simulink model "management_2_sources_21_03_2023_flc_9aa"  (R2016b)
settings: Solver=FixedStepAuto  StartTime=0.0  StopTime=25  RelTol=1e-3
undefined symbols (not defined in the file): DiscIntNeverNeededParam, sigbuilder_block
libraries: powerlib x31, simulink x8, powerlib_meascontrol x7, fuzblock x1, powerlib_extras x1
(part 2 of 2)

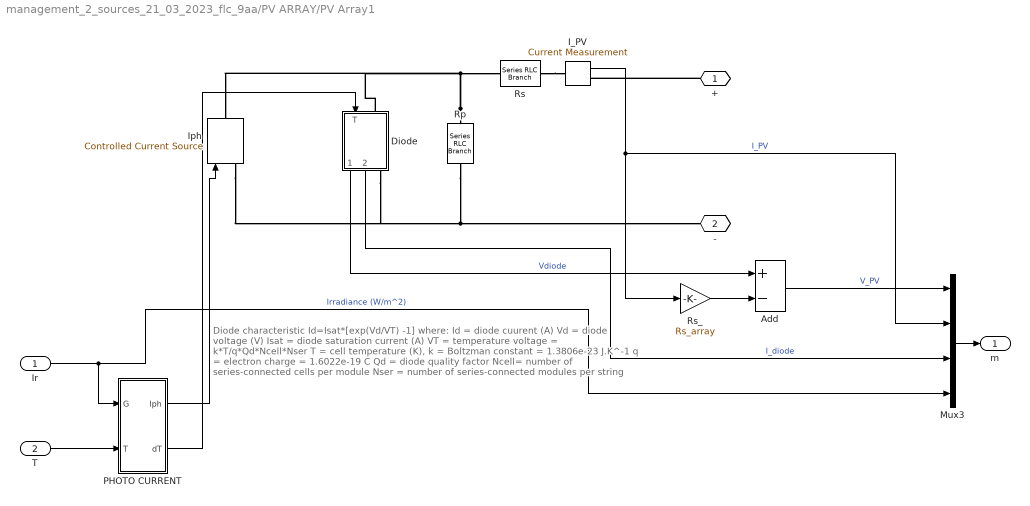
== system management_2_sources_21_03_2023_flc_9aa/PV ARRAY/PV Array1 ==
  note: Diode characteristic
      |    Id=Isat*[exp(Vd/VT) -1]
      |
      | where:
      |    Id = diode cuurent (A)
      |    Vd = diode voltage (V)
      |  Isat = diode saturation current (A)
      |    VT = temperature voltage = k*T/q*Qd*Ncell*Nser
      |
      |     T = cell temperature (K),
      |     k = Boltzman constant = 1.3806e-23 J.K^-1
      |     q = electron charge = 1.6022e-19 C
      |    Qd = diode quality factor
      |  Ncell= number of series-connected cells per module
      |  Nser = number of series-connected modules per string
  Ir : Inport
  T : Inport  Port=2
  Add : Sum  Inputs=+-
  Diode : Subsystem
      mask Display:
      | plot(-75,-50,100,150, [-15 -15 43 -15 -15 -75],[50 8 50 92 50 50], ...
      |     [43 43],[8 94],[100 43], [50 50])
  I_PV : powerlib/Measurements/Current Measurement  PhasorSimulation=off  OutputType=Complex  PSBequivalent=0
  Iph : powerlib/Electrical Sources/Controlled Current Source  Initialize=on  Source_Type=AC  Amplitude=0  Phase=0  Frequency=0  Measurements=None
  Mux3 : Mux
  PHOTO CURRENT : Subsystem
  Rp : powerlib/Elements/Series RLC Branch  LConnTagsString=__new0  RConnTagsString=__new0  BranchType=R  Resistance=Rp_array  Inductance=1e-3  SetiL0=off  InitialCurrent=0  Capacitance=1e-6  Setx0=off  InitialVoltage=0  Measurements=Branch current
  Rs : powerlib/Elements/Series RLC Branch  LConnTagsString=__new0  RConnTagsString=__new0  BranchType=R  Resistance=Rs_array  Inductance=1e-3  SetiL0=off  InitialCurrent=0  Capacitance=1e-6  Setx0=off  InitialVoltage=0  Measurements=None
  Rs_ : Gain  Gain=Rs_array
  + : PMIOPort  Port=1  Side=Right
  - : PMIOPort  Port=2  Side=Right
  m : Outport
  wires:
  Diode/2(Idiode) -> Mux3/3  "I_diode"
  Add/1 -> Mux3/1  "V_PV"
  I_PV/1 -> Mux3/2, Rs_/1  "I_PV"
  Rs_/1 -> Add/2
  Diode/1(Vdiode) -> Add/1  "Vdiode"
  Ir/1 -> Mux3/4, PHOTO CURRENT/1(G)  "Irradiance (W/m^2)"
  PHOTO CURRENT/1("Iph ") -> Iph/1
  T/1 -> PHOTO CURRENT/2(T)
  PHOTO CURRENT/2(dT) -> Diode/1(T)
  Mux3/1 -> m/1
  connections:
  +/RConn1 -- I_PV/RConn1
  Rs/LConn1 -- I_PV/LConn1
  Rp/LConn1 -- Rs/RConn1 -- Iph/RConn1 -- Diode/LConn1
  Rp/RConn1 -- -/RConn1 -- Diode/RConn1 -- Iph/LConn1

== system management_2_sources_21_03_2023_flc_9aa/PV ARRAY/boost converter ==
  pwm : Inport
  C1 : powerlib/Elements/Series RLC Branch  LConnTagsString=__new0  RConnTagsString=__new0  BranchType=C  Resistance=1.0  Inductance=1.0  SetiL0=off  InitialCurrent=0  Capacitance=100e-6  Setx0=off  InitialVoltage=0  Measurements=None
  Diode1 : powerlib/Power Electronics/Diode  Ron=1e-4  Lon=0  Vf=0  IC=0  UseSnubber=off  Rs=inf  Cs=inf  Measurements=off
  IGBT1 : powerlib/Power Electronics/IGBT  Ron=0.001  Lon=0  Vf=0  Tf=0  Tt=0  IC=0  Rs=1e5  Cs=inf  Measurements=off
  L1 : powerlib/Elements/Series RLC Branch  LConnTagsString=__new0  RConnTagsString=__new0  BranchType=RL  Resistance=0.005  Inductance=5e-3  SetiL0=off  InitialCurrent=0  Capacitance=1e-6  Setx0=off  InitialVoltage=0  Measurements=None
  out + : PMIOPort  Port=1  Side=Right
  in + : PMIOPort  Port=2  Side=Left
  in - : PMIOPort  Port=3  Side=Left
  out - : PMIOPort  Port=4  Side=Right
  wires:
  pwm/1 -> IGBT1/1
  connections:
  C1/LConn1 -- in +/RConn1 -- L1/LConn1
  IGBT1/LConn1 -- L1/RConn1 -- Diode1/LConn1
  out +/RConn1 -- Diode1/RConn1
  C1/RConn1 -- in -/RConn1 -- out -/RConn1 -- IGBT1/RConn1

== system management_2_sources_21_03_2023_flc_9aa/Subsystem2/Dashboard Scope ==

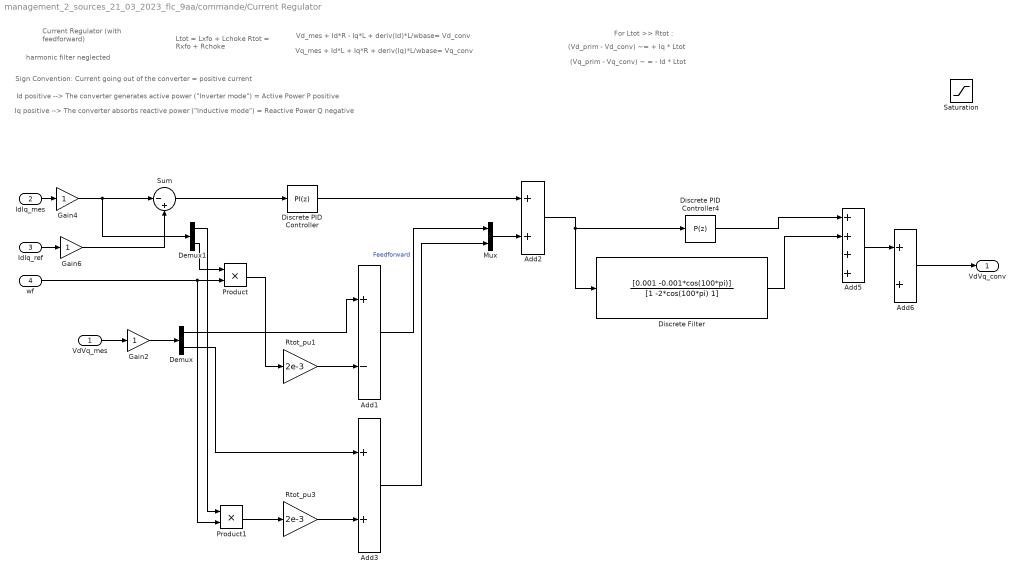
== system management_2_sources_21_03_2023_flc_9aa/commande/Current Regulator ==
  note: harmonic filter neglected
  note: Vd_mes + Id*R - Iq*L + deriv(Id)*L/wbase= Vd_conv
  note: Vq_mes + Id*L + Iq*R + deriv(Iq)*L/wbase= Vq_conv
  note: Current Regulator
      | (with feedforward)
  note: Sign Convention: Current going out of the converter = positive current
  note: Iq positive --> The converter absorbs reactive power ("Inductive mode") = Reactive Power Q negative
  note: Id positive --> The converter generates active power ("Inverter mode") = Active Power P positive
  note: Ltot = Lxfo + Lchoke
      | Rtot = Rxfo + Rchoke
  note: (Vd_prim - Vd_conv) ~= + Iq * Ltot
  note: (Vq_prim - Vq_conv) ~ = - Id * Ltot
  note: For Ltot >> Rtot :
  VdVq_mes : Inport  PortDimensions=2
  IdIq_mes : Inport  Port=2  PortDimensions=2
  IdIq_ref : Inport  Port=3  PortDimensions=2
  wf : Inport  Port=4  PortDimensions=1
  Add1 : Sum  Inputs=+-
  Add2 : Sum
  Add3 : Sum
  Add5 : Sum  Inputs=++++
  Add6 : Sum
  Demux : Demux  Outputs=2
  Demux1 : Demux  Outputs=2
  Discrete Filter : DiscreteFilter  Numerator=[0.001 -0.001*cos(100*pi)]  Denominator=[1 -2*cos(100*pi) 1]  SampleTime=1e-5
  Discrete PID Controller : simulink/Continuous/PID Controller  Controller=PI  TimeDomain=Discrete-time  SampleTime=-1  IntegratorMethod=Trapezoidal  FilterMethod=Forward Euler  Form=Parallel  UseFilter=on  ControllerParametersSource=internal  P=24  I=12  D=0  N=100  InitialConditionSource=internal  InitialConditionForIntegrator=0  InitialConditionForFilter=0  ExternalReset=none  LimitOutput=on  UpperSaturationLimit=1000  LowerSaturationLimit=-1000  LinearizeAsGain=off  AntiWindupMode=none  Kb=1  TrackingMode=off  Kt=1  PParamMin=[]  PParamMax=[]  IParamMin=[]  IParamMax=[]  DParamMin=[]  DParamMax=[]  NParamMin=[]  NParamMax=[]  KbParamMin=[]  KbParamMax=[]  KtParamMin=[]  KtParamMax=[]  POutMin=[]  POutMax=[]  IOutMin=[]  IOutMax=[]  DOutMin=[]  DOutMax=[]  NOutMin=[]  NOutMax=[]  KbOutMin=[]  KbOutMax=[]  KtOutMin=[]  KtOutMax=[]  IntegratorOutMin=[]  IntegratorOutMax=[]  FilterOutMin=[]  FilterOutMax=[]  SumOutMin=[]  SumOutMax=[]  SumI1OutMin=[]  SumI1OutMax=[]  SumI2OutMin=[]  SumI2OutMax=[]  SumI3OutMin=[]  SumI3OutMax=[]  SumDOutMin=[]  SumDOutMax=[]  SaturationOutMin=[]  SaturationOutMax=[]  IntegratorContinuousStateAttributes=''  IntegratorStateMustResolveToSignalObject=off  IntegratorRTWStateStorageClass=Auto  FilterContinuousStateAttributes=''  FilterStateMustResolveToSignalObject=off  FilterRTWStateStorageClass=Auto  DifferentiatorICPrevScaledInput=0  DifferentiatorOutMin=[]  DifferentiatorOutMax=[]
  Discrete PID Controller4 : simulink/Continuous/PID Controller  Controller=P  TimeDomain=Discrete-time  SampleTime=-1  IntegratorMethod=Trapezoidal  FilterMethod=Forward Euler  Form=Parallel  UseFilter=on  ControllerParametersSource=internal  P=60  I=12  D=0  N=100  InitialConditionSource=internal  InitialConditionForIntegrator=0  InitialConditionForFilter=0  ExternalReset=none  LimitOutput=on  UpperSaturationLimit=1000  LowerSaturationLimit=-1000  LinearizeAsGain=off  AntiWindupMode=none  Kb=1  TrackingMode=off  Kt=1  PParamMin=[]  PParamMax=[]  IParamMin=[]  IParamMax=[]  DParamMin=[]  DParamMax=[]  NParamMin=[]  NParamMax=[]  KbParamMin=[]  KbParamMax=[]  KtParamMin=[]  KtParamMax=[]  POutMin=[]  POutMax=[]  IOutMin=[]  IOutMax=[]  DOutMin=[]  DOutMax=[]  NOutMin=[]  NOutMax=[]  KbOutMin=[]  KbOutMax=[]  KtOutMin=[]  KtOutMax=[]  IntegratorOutMin=[]  IntegratorOutMax=[]  FilterOutMin=[]  FilterOutMax=[]  SumOutMin=[]  SumOutMax=[]  SumI1OutMin=[]  SumI1OutMax=[]  SumI2OutMin=[]  SumI2OutMax=[]  SumI3OutMin=[]  SumI3OutMax=[]  SumDOutMin=[]  SumDOutMax=[]  SaturationOutMin=[]  SaturationOutMax=[]  IntegratorContinuousStateAttributes=''  IntegratorStateMustResolveToSignalObject=off  IntegratorRTWStateStorageClass=Auto  FilterContinuousStateAttributes=''  FilterStateMustResolveToSignalObject=off  FilterRTWStateStorageClass=Auto  DifferentiatorICPrevScaledInput=0  DifferentiatorOutMin=[]  DifferentiatorOutMax=[]
  Gain2 : Gain
  Gain4 : Gain
  Gain6 : Gain
  Mux : Mux  Inputs=2
  Product : Product
  Product1 : Product
  Rtot_pu1 : Gain  Gain=2e-3  SaturateOnIntegerOverflow=on  OutDataTypeStr=Inherit: Same as input  ParamDataTypeStr=Inherit: Same as input
  Rtot_pu3 : Gain  Gain=2e-3  SaturateOnIntegerOverflow=on  OutDataTypeStr=Inherit: Same as input  ParamDataTypeStr=Inherit: Same as input
  Saturation : Saturate  UpperLimit=5  LowerLimit=-5
  Sum : Sum  Inputs=|-+
  VdVq_conv : Outport
  wires:
  Mux/1 -> Add2/2
  IdIq_ref/1 -> Gain6/1
  Add1/1 -> Mux/1  "Feedforward"
  Add3/1 -> Mux/2
  IdIq_mes/1 -> Gain4/1
  Demux/1 -> Add1/1
  Rtot_pu1/1 -> Add1/2
  Demux/2 -> Add3/1
  Rtot_pu3/1 -> Add3/2
  VdVq_mes/1 -> Gain2/1
  Discrete PID Controller/1 -> Add2/1
  Product/1 -> Rtot_pu1/1
  Demux1/2 -> Product/1
  Product1/1 -> Rtot_pu3/1
  Demux1/1 -> Product1/1
  wf/1 -> Product1/2, Product/2
  Gain4/1 -> Demux1/1, Sum/1
  Gain2/1 -> Demux/1
  Gain6/1 -> Sum/2
  Sum/1 -> Discrete PID Controller/1
  Discrete PID Controller4/1 -> Add5/1
  Add5/1 -> Add6/1
  Add2/1 -> Discrete Filter/1, Discrete PID Controller4/1
  Add6/1 -> VdVq_conv/1
  Discrete Filter/1 -> Add5/2

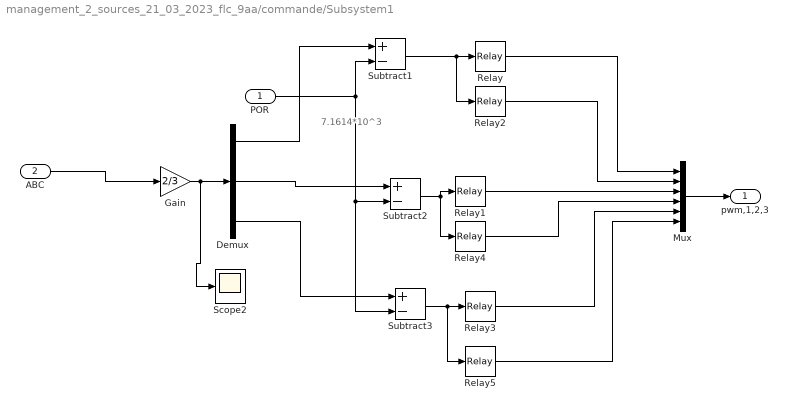
== system management_2_sources_21_03_2023_flc_9aa/commande/Subsystem1 ==
  note: 7.1614*10^3
  POR : Inport
  ABC : Inport  Port=2
  Demux : Demux  Outputs=3
  Gain : Gain  Gain=2/3
  Mux : Mux  Inputs=6
  Relay : Relay
  Relay1 : Relay
  Relay2 : Relay  OnOutputValue=0  OffOutputValue=1
  Relay3 : Relay
  Relay4 : Relay  OnOutputValue=0  OffOutputValue=1
  Relay5 : Relay  OnOutputValue=0  OffOutputValue=1
  Scope2 : Scope
  Subtract1 : Sum  Inputs=+-
  Subtract2 : Sum  Inputs=+-
  Subtract3 : Sum  Inputs=+-
  pwm,1,2,3 : Outport
  wires:
  POR/1 -> Subtract2/2, Subtract3/2, Subtract1/2
  Subtract1/1 -> Relay2/1, Relay/1
  Relay/1 -> Mux/1
  Subtract2/1 -> Relay1/1, Relay4/1
  Mux/1 -> pwm,1,2,3/1
  Gain/1 -> Scope2/1, Demux/1
  Subtract3/1 -> Relay5/1, Relay3/1
  Relay2/1 -> Mux/2
  Relay1/1 -> Mux/3
  Relay4/1 -> Mux/4
  Relay3/1 -> Mux/5
  Relay5/1 -> Mux/6
  Demux/1 -> Subtract1/1
  Demux/2 -> Subtract2/1
  Demux/3 -> Subtract3/1
  ABC/1 -> Gain/1

== system management_2_sources_21_03_2023_flc_9aa/PV ARRAY/Boost Converter Control (MPPT)/Pulse Generator ==
  D : Inport
  Relational Operator : RelationalOperator  Operator=<=  OutDataTypeStr=boolean  RndMeth=Nearest
  Repeating Sequence : simulink/Sources/Repeating Sequence  rep_seq_t="[0  1/Freq]"  rep_seq_y=[0 1]
  Pulses : Outport
  wires:
  D/1 -> Relational Operator/2
  Relational Operator/1 -> Pulses/1
  Repeating Sequence/1 -> Relational Operator/1

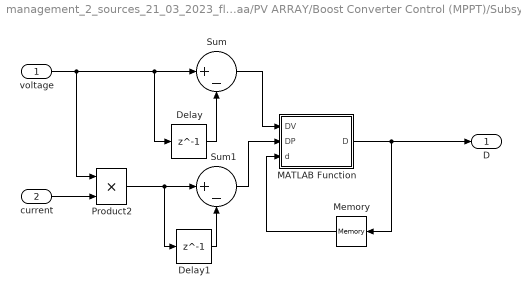
== system management_2_sources_21_03_2023_flc_9aa/PV ARRAY/Boost Converter Control (MPPT)/Subsystem2 ==
  "voltage " : Inport
  "current " : Inport  Port=2
  Delay : Delay  DelayLength=1  InitialCondition=0
  Delay1 : Delay  DelayLength=1  InitialCondition=0
  MATLAB Function : MATLAB Function  TreatAsAtomicUnit=on
  Memory : Memory  X0=0.7
  Product2 : Product
  Sum : Sum  Inputs=|+-
  Sum1 : Sum  Inputs=|+-
  D : Outport
  wires:
  Delay/1 -> Sum/2
  Delay1/1 -> Sum1/2
  "voltage "/1 -> Product2/1, Delay/1, Sum/1
  "current "/1 -> Product2/2
  Sum1/1 -> MATLAB Function/2(DP)
  Sum/1 -> MATLAB Function/1(DV)
  Product2/1 -> Delay1/1, Sum1/1
  MATLAB Function/1(D) -> Memory/1, D/1
  Memory/1 -> MATLAB Function/3(d)

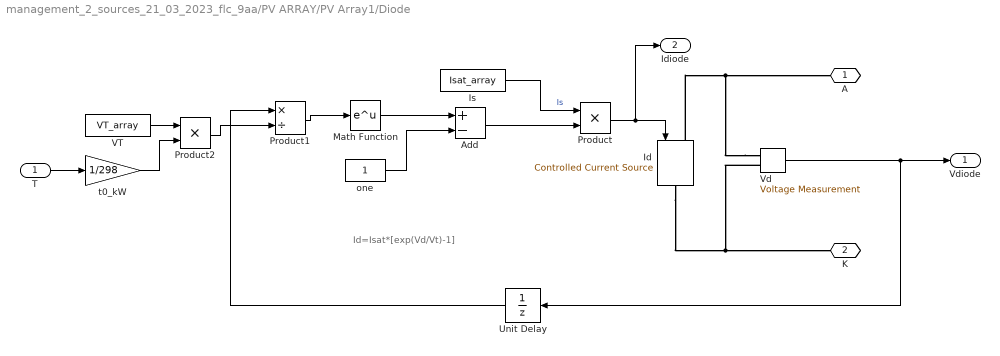
== system management_2_sources_21_03_2023_flc_9aa/PV ARRAY/PV Array1/Diode ==
  note: Id=Isat*[exp(Vd/Vt)-1]
  T : Inport
  Add : Sum  Inputs=+-
  Id : powerlib/Electrical Sources/Controlled Current Source  Initialize=on  Source_Type=AC  Amplitude=0  Phase=0  Frequency=0  Measurements=None
  Is : Constant  Value=Isat_array
  Math Function : Math  SaturateOnIntegerOverflow=on
  Product : Product  RndMeth=Zero
  Product1 : Product  Inputs=*/  RndMeth=Zero
  Product2 : Product  RndMeth=Zero
  Unit Delay : UnitDelay  SampleTime=-1
  VT : Constant  Value=VT_array
  Vd : powerlib/Measurements/Voltage Measurement  PhasorSimulation=off  OutputType=Complex  PSBequivalent=0
  one : Constant
  t0_kW : Gain  Gain=1/298
  A : PMIOPort  Port=1  Side=Left
  K : PMIOPort  Port=2  Side=Right
  Vdiode : Outport
  Idiode : Outport  Port=2
  wires:
  Product/1 -> Idiode/1, Id/1
  Vd/1 -> Vdiode/1, Unit Delay/1
  Is/1 -> Product/1  "Is"
  Product1/1 -> Math Function/1
  one/1 -> Add/2
  Add/1 -> Product/2
  Unit Delay/1 -> Product1/1
  Math Function/1 -> Add/1
  VT/1 -> Product2/1
  T/1 -> t0_kW/1
  Product2/1 -> Product1/2
  t0_kW/1 -> Product2/2
  connections:
  Id/RConn1 -- K/RConn1 -- Vd/LConn2
  Vd/LConn1 -- A/RConn1 -- Id/LConn1

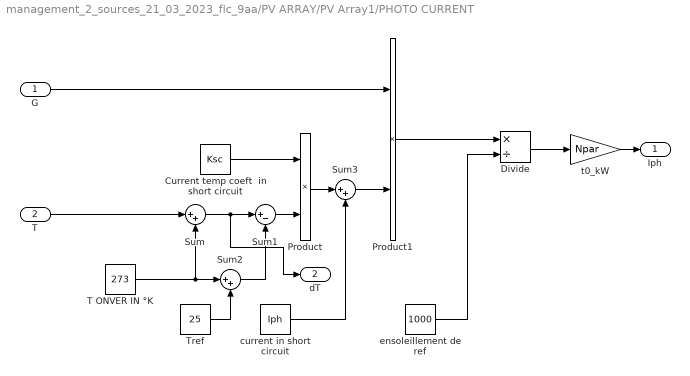
== system management_2_sources_21_03_2023_flc_9aa/PV ARRAY/PV Array1/PHOTO CURRENT ==
  G : Inport
  T : Inport  Port=2
  Current temp coeft  in short circuit : Constant  Value=Ksc
  Divide : Product  Inputs=*/
  Product : Product
  Product1 : Product
  Sum : Sum  Inputs=|++
  Sum1 : Sum  Inputs=|+-
  Sum2 : Sum  Inputs=|++
  Sum3 : Sum  Inputs=|++
  "T ONVER IN °K " : Constant  Value=273
  Tref : Constant  Value=25
  current in short circuit : Constant  Value=Iph
  ensoleillement de ref : Constant  Value=1000
  t0_kW : Gain  Gain=Npar
  "Iph " : Outport
  dT : Outport  Port=2
  wires:
  Sum2/1 -> Sum1/2
  Product/1 -> Sum3/1
  Sum3/1 -> Product1/2
  ensoleillement de ref/1 -> Divide/2
  current in short circuit/1 -> Sum3/2
  G/1 -> Product1/1
  Current temp coeft  in short circuit/1 -> Product/1
  Tref/1 -> Sum2/2
  Sum/1 -> dT/1, Sum1/1
  Sum1/1 -> Product/2
  Product1/1 -> Divide/1
  "T ONVER IN °K "/1 -> Sum2/1, Sum/2
  Divide/1 -> t0_kW/1
  T/1 -> Sum/1
  t0_kW/1 -> "Iph "/1

== matlab function management_2_sources_21_03_2023_flc_9aa/PV ARRAY/Boost Converter Control (MPPT)/Subsystem2/MATLAB Function ==
  data: DV input; DP input; D output; d input
function D = fcn(DV,DP,d)
D=0;p=0.001;
    if(DP>0)
        if(DV>0)
         D=d-p;
        else
            D=d+p;
        end
    end
    if(DP<0)
        if(DV>0)
         D=d+p;
        else
            D=d-p;
      
        end
    end
     if DP==0
        D=d;
    end 
    if D>1
        D=1;
    end 
    if D<0
        D=0;
    end
end
